simulink model "METI_TRAMI_Thermal_ver01_Jmaab_2018b_Intg"  (R2018b)
settings: Solver=ode8  StartTime=0  StopTime=end_time  FixedStep=sampling_time  RelTol=1e-3
PreLoadFcn:
  | METI_TRAMI_Thermal_ver01_Jmaab_PreLoad;
values from neighbouring files (symbols this model uses):
  degC2K = 273.15    [METI_TRAMI_Thermal_ver01_Jmaab_PreLoad.m]    (also in init_setting_METI.m)
  K2degC = -273.15    [METI_TRAMI_Thermal_ver01_Jmaab_PreLoad.m]    (also in init_setting_METI.m)
undefined symbols (not defined in the file or in its folder): ACC_D_Gain, ACC_I_Gain, ACC_P_Gain, ALT_CNT_ALT_OFF_RPM_HYS_rpm, ALT_CNT_ALT_ON_RPM_HYS_rpm, ALT_CNT_Alter_V_BASE_V, ALT_CNT_Alter_V_Kaisei_V, ALT_CNT_flag_disable_kaisei, ALT_CNT_V_Battely_Kudo_V, ALT_PNT_ALT_GDCurrent_A, ALT_PNT_ALT_GDVolt_V, ALT_PNT_Alter_limit_Current_V_table, ALT_PNT_Alter_limit_Current_V_table_x_rpm, ALT_PNT_Alter_trq_Nm_map, ALT_PNT_Alter_trq_Nm_map_x_rpm, ALT_PNT_Alter_trq_Nm_map_y_Current_A, ALT_PNT_Alter_trq_Nm_map_z_Volt_tgt_V, ALT_PNT_eta_pulley_alt, ALT_PNT_Gain_Alt_v_del, ALT_PNT_ratio_pulley_alt, ALT_PNT_Tau_Alternator_V_tgt_s, ALT_PNT_trq_alter_output_LL_Nm, BK_PNT_Pow_UL, BK_PNT_Tau_brake, Brk_LL, Brk_PGain, Brk_UL, BT_PNT_Lo_Capa_lo_batt_F, BT_PNT_Lo_ocv_SOC_lo_batt_OCV_V_table, BT_PNT_Lo_ocv_SOC_lo_batt_OCV_V_table_x_SOC, BT_PNT_Lo_R_lo_batt_ohm, BT_PNT_Lo_SOC_MAX_lo_batt, BT_PNT_Lo_SOC_MIN_lo_batt, BT_PNT_Lo_SOC_START_lo_batt, BT_PNT_Lo_V_start_ocv, DF_PNT_DF_gear, DF_PNT_DFBlock2DFAir_Heat_Resi_KpW, DF_PNT_DFBlock_Heat_Capa_JpK, DF_PNT_DFBlock_Temp_ini_degC, DF_PNT_DFOil2DFBlock_Heat_Resi_KpW, DF_PNT_DFOil_Heat_Capa_JpK, DF_PNT_DFOil_Temp_ini_degC, DF_PNT_Driveshaft_damper, DF_PNT_Driveshaft_delta_radps_LL, DF_PNT_Driveshaft_delta_radps_UL, DF_PNT_Driveshaft_spring, DF_PNT_eta_DF, DF_PNT_Outtemp_degC, DF_PNT_TMBlock2DFBlock_Heat_Resi_KpW, Driver_Brake_Const1, Driver_Brake_Const3, Driver_Brake_Switch_Const2, Driver_Brk_sh, drivmode_ACC, drivmode_CONST, drivmode_GensokuKaisei, drivmode_GensokuRikko, drivmode_STOP, EL_PNT_R_bodyelec_lo_ohm, ENG_CNT_acc_idlestop ... (+139)
libraries: METI_Lib_vehicle_model x33, simulink x7, AZAPA_Lib_vehicle_model x1
(part 4 of 4)

== system METI_TRAMI_Thermal_ver01_Jmaab_2018b_Intg/Driver/Driver_TRAMI/Driver2/Caliculate_Opeining_Accel/FF/Cal_M_ENG_jiku2 ==
  note: 軸トルクマップ
  FF_trq_accel_Nm : Inport
  pre_n_eng_rpm : Inport  Port=2
  2-D Lookup Table : Lookup_n-D  BreakpointsForDimension1=ENG_trq_rev  BreakpointsForDimension2=ENG_rpm  Table=ENG_throttle_rev  ExtrapMethod=Clip  UseLastTableValue=on  RndMeth=Simplest  InputSameDT=on
  2-D Lookup Table1 : Lookup_n-D  BreakpointsForDimension1=ENG_PNT_trq_Nm_map_y_throttle  BreakpointsForDimension2=ENG_PNT_trq_Nm_map_x_rpm  Table=ENG_PNT_trq_Nm_map  ExtrapMethod=Clip  UseLastTableValue=on  RndMeth=Simplest  InputSameDT=on
  Constant : Constant  Value=0
  Subsystem : Subsystem
  Sum : Sum  Inputs=|++
  FF_open_accel_per : Outport
  wires:
  FF_trq_accel_Nm/1 -> Sum/1
  2-D Lookup Table/1 -> Subsystem/1(In1)
  pre_n_eng_rpm/1 -> 2-D Lookup Table/2, 2-D Lookup Table1/2
  Constant/1 -> 2-D Lookup Table1/1
  Sum/1 -> 2-D Lookup Table/1
  2-D Lookup Table1/1 -> Sum/2
  Subsystem/1(Out1) -> FF_open_accel_per/1

== system METI_TRAMI_Thermal_ver01_Jmaab_2018b_Intg/Driver/Driver_TRAMI/Driver2/Caliculate_Opeining_Accel/FF/Inertial_Resistance ==
  V_tgt : Inport
  Constant : Constant  Value=M
  Derivative : Derivative
  Divide : Product  OutDataTypeStr=Inherit: Same as first input
  F_Inertia : Outport
  wires:
  Constant/1 -> Divide/2
  Derivative/1 -> Divide/1
  Divide/1 -> F_Inertia/1
  V_tgt/1 -> Derivative/1

== system METI_TRAMI_Thermal_ver01_Jmaab_2018b_Intg/Driver/Driver_TRAMI/Driver2/Caliculate_Opeining_Accel/FF/Rolling_Resistance ==
  note: 20151211修正
      |
      | 空気抵抗と表現を統一する、ため
      | -1のGainを削除
  V_tgt : Inport
  cal_roll_resi1 : METI_Lib_vehicle_model/vehicle_model/cal_roll_resi  Myu_tire=myu  Vehicle_Mass=M  Gravi_acc=g
      settings: SourceProductName=The database C:\Users\k-uekata\AppData\Roaming\MathWorks\MATLAB\R2018b\slblocks_master.db is locked, or a table in the database is locked. (database is locked)
  F_rollresi : Outport
  wires:
  V_tgt/1 -> cal_roll_resi1/1
  cal_roll_resi1/1 -> F_rollresi/1

== system METI_TRAMI_Thermal_ver01_Jmaab_2018b_Intg/Vehicle/CNT/ENG_CNT/ENG_Cntrl/Caliculate_Idle_Speed/Subsystem ==
  del_omg_engine : Inport
  flag_idle_fb : Inport  Port=2
  Gain : Gain  Gain=ENG_CNT_gain_p_per_isc
  Logical Operator1 : Logic  Operator=NOT  AllPortsSameDT=off  OutDataTypeStr=boolean
  Memory : Memory  InitialCondition=4
  Saturation : Saturate  UpperLimit=ENG_CNT_per_isc_max  LowerLimit=ENG_CNT_per_isc_min
  Switch : Switch  Criteria=u2 > Threshold  Threshold=0.5
  per_isc_[%] : Outport
  wires:
  Logical Operator1/1 -> Switch/2
  del_omg_engine/1 -> Gain/1
  Saturation/1 -> Memory/1, per_isc_[%]/1
  Memory/1 -> Switch/1
  Gain/1 -> Switch/3
  flag_idle_fb/1 -> Logical Operator1/1
  Switch/1 -> Saturation/1

== system METI_TRAMI_Thermal_ver01_Jmaab_2018b_Intg/Vehicle/CNT/ENG_CNT/ENG_Cntrl/Caliculate_Idle_Speed/Subsystem1 ==
  note: アイドル回転数時のFB
  omg_tgt_idle : Inport
  n_eng_rpm : Inport  Port=2
  per_throttle_base : Inport  Port=3
  flag_Lockup : Inport  Port=4
  flag_IdleStop : Inport  Port=5
  Logical Operator : Logic  Operator=OR  AllPortsSameDT=off  OutDataTypeStr=boolean
  Logical Operator1 : Logic  Operator=NOT  AllPortsSameDT=off  OutDataTypeStr=boolean
  Logical Operator2 : Logic  Inputs=3  AllPortsSameDT=off  OutDataTypeStr=boolean
  Logical Operator3 : Logic  Operator=NOT  AllPortsSameDT=off  OutDataTypeStr=boolean
  Logical Operator4 : Logic  Operator=NOT  AllPortsSameDT=off  OutDataTypeStr=boolean
  Logical Operator5 : Logic  AllPortsSameDT=off  OutDataTypeStr=boolean
  Relational Operator : RelationalOperator  Operator=<  OutDataTypeStr=boolean  RndMeth=Nearest
  Relational Operator2 : RelationalOperator  Operator=>  OutDataTypeStr=boolean  RndMeth=Nearest
  per_throttle_isc_fb : Constant  Value=ENG_CNT_per_throttle_isc_fb
  flag_idle_fb : Outport
  wires:
  Logical Operator/1 -> flag_idle_fb/1
  Logical Operator4/1 -> Logical Operator5/2
  flag_IdleStop/1 -> Logical Operator4/1
  n_eng_rpm/1 -> Relational Operator2/2
  omg_tgt_idle/1 -> Relational Operator2/1
  Logical Operator2/1 -> Logical Operator/1
  Logical Operator3/1 -> Logical Operator2/3
  flag_Lockup/1 -> Logical Operator3/1
  Logical Operator5/1 -> Logical Operator/2
  Logical Operator1/1 -> Logical Operator2/2
  Relational Operator/1 -> Logical Operator5/1, Logical Operator1/1
  Relational Operator2/1 -> Logical Operator2/1
  per_throttle_isc_fb/1 -> Relational Operator/2
  per_throttle_base/1 -> Relational Operator/1

== system METI_TRAMI_Thermal_ver01_Jmaab_2018b_Intg/Vehicle/CNT/TM_CNT/TM_CNT/TM_CNT/TM_Ctrl ==
  v_VL_PNT_kmph : Inport
  n_TM_PNT_rpm : Inport  Port=2
  T_TMTH_PNT_CVTF_degC : Inport  Port=3
  T_ENGTH_PNT_Coolant_degC : Inport  Port=4
  open_throttle_per : Inport  Port=5
  CVT_ECU : Subsystem
  K->degC : Subsystem  Commented=through
  K->degC1 : Subsystem  Commented=through
  LockupClutch_ECU : Subsystem
  Memory{,1..4} (5 alike) : Memory  Commented=through
  Signal Specification : SignalSpecification
  Signal Specification1 : SignalSpecification
  WarmerECU : Subsystem
  flag_Lockup : Outport
  omg_Slip_rpm : Outport  Port=2
  ratio_CVT : Outport  Port=3
  R_CVTF_warmer_tgt_KpW : Outport  Port=4
  tag scope: tScope_CVTratio=scoped, tScope_Luckup=scoped
  wires:
  CVT_ECU/1(ratio_CVT) -> Signal Specification1/1, ratio_CVT/1  "ratio_CVT"
  LockupClutch_ECU/1(flag_Lockup) -> Signal Specification/1, flag_Lockup/1  "flag_Lockup"
  LockupClutch_ECU/2(omg_Slip_rpm) -> omg_Slip_rpm/1  "omg_Slip_rpm"
  open_throttle_per/1 -> Memory1/1
  Memory/1 -> LockupClutch_ECU/1(v_vehicle)
  Memory1/1 -> CVT_ECU/1(per_throttle), LockupClutch_ECU/2(per_throttle)
  Memory2/1 -> CVT_ECU/2(omg_pera)
  n_TM_PNT_rpm/1 -> Memory2/1
  v_VL_PNT_kmph/1 -> Memory/1
  T_TMTH_PNT_CVTF_degC/1 -> Memory3/1
  T_ENGTH_PNT_Coolant_degC/1 -> Memory4/1
  Memory3/1 -> K->degC/1(K)
  Memory4/1 -> K->degC1/1(K)
  WarmerECU/1(R_CVTF_warmer_tgt_KpW) -> R_CVTF_warmer_tgt_KpW/1  "R_CVTF_warmer_tgt_KpW"
  K->degC/1(degC) -> WarmerECU/1(T_TMTH_PNT_CVTF_dC)
  K->degC1/1(degC) -> WarmerECU/2(T_ENG_Coolant_dC)
  Signal Specification/1 -> [tScope_Luckup]  "tScope_Luckup"
  Signal Specification1/1 -> [tScope_CVTratio]  "tScope_CVTratio"

== system METI_TRAMI_Thermal_ver01_Jmaab_2018b_Intg/Vehicle/PTTH/DTTH_PNT/DTTH_PNT/DTTH_PNT/DFTH_PNT ==
  note: T/Mブロックから
      | 受け取る熱量
  note: DFオイルの
      | 熱容量
  note: DFブロックの
      | 熱容量
  note: DFの損失が
      | DFオイルへの熱量
  note: エネルギーの
      | 向きの定義（仮）
      | →→→
  note: エネルギーの
      | 向きの定義（仮）
      | →→→
  note: エネルギーの
      | 向きの定義（仮）
      | →→→
  note: エネルギーの
      | 向きの定義（仮）
      | →→→
  note: エネルギーの
      | 向きの定義（仮）
      | →→→
  T_DF_Block_K : Inport
  PHI_DF_PNT_W : Inport  Port=2
  T_ATM_PNT_DF_K : Inport  Port=3
  DFBlock_Heat_Capacity : Subsystem
  DFOil2DFBlock_Heat_Resistance : Subsystem
  DFOil_Heat_Capacity : Subsystem
  ENGBlock2Air_Heat_Resistance : Subsystem
  TMBlock2DFBlock_Heat_Resistance : Subsystem
  Terminator : Terminator
  PHI_DF_Block_W : Outport
  PHI_DFTH_PNT_W : Outport  Port=2
  T_DFBlock_K : Outport  Port=3
  wires:
  DFOil_Heat_Capacity/1(T_DFOil2_K) -> DFOil2DFBlock_Heat_Resistance/1(T_DFOil_Resi2_K)
  DFOil2DFBlock_Heat_Resistance/1(PHI_DFOil_Resi2_W) -> DFOil_Heat_Capacity/1(PHI_DFOil2_W)
  DFBlock_Heat_Capacity/3(T_DFBlock1_K) -> DFOil2DFBlock_Heat_Resistance/2(T_DFBlock_Resi_K)
  DFOil2DFBlock_Heat_Resistance/2(PHI_DFBlock_Resi_W) -> DFBlock_Heat_Capacity/3(PHI_DFBlock1_W)
  ENGBlock2Air_Heat_Resistance/1(PHI_DFBlock_Resi_W) -> DFBlock_Heat_Capacity/1(PHI_DFBlock3_W)
  DFBlock_Heat_Capacity/2(T_DFBlock3_K) -> ENGBlock2Air_Heat_Resistance/1(T_DFBlock_Resi_K)
  T_ATM_PNT_DF_K/1 -> ENGBlock2Air_Heat_Resistance/2(T_DF_Air_Resi_K)
  ENGBlock2Air_Heat_Resistance/2(PHI_DF_Air_Resi_W) -> PHI_DFTH_PNT_W/1  "PHI_DFTH_PNT_W"
  T_DF_Block_K/1 -> TMBlock2DFBlock_Heat_Resistance/2(T_TMBlock_Resi_K)
  TMBlock2DFBlock_Heat_Resistance/2(PHI_TMBlock_Resi_W) -> PHI_DF_Block_W/1  "PHI_DF_Block_W"
  TMBlock2DFBlock_Heat_Resistance/1(PHI_DFBlock_Resi_W) -> DFBlock_Heat_Capacity/2(PHI_DFBlock2_W)
  DFBlock_Heat_Capacity/1(T_DFBlock2_K) -> T_DFBlock_K/1, TMBlock2DFBlock_Heat_Resistance/1(T_DFBlock_Resi_K)  "T_DFBlock_K"
  DFOil_Heat_Capacity/2(T_DFOil1_K) -> Terminator/1
  PHI_DF_PNT_W/1 -> DFOil_Heat_Capacity/2(PHI_DFOil1_W)

== system METI_TRAMI_Thermal_ver01_Jmaab_2018b_Intg/Vehicle/PTTH/DTTH_PNT/DTTH_PNT/DTTH_PNT/TMTH_PNT ==
  note: CVTFの
      | 熱容量
  note: T/Mブロックの
      | 熱容量
  note: DFブロックへ
      | 放熱する熱量
  note: エンジンブロックから
      | 受け取る熱量
  note: CVTFからエンジン冷却水へ
      | 放熱する熱量
  note: T/Mの入力-出力が
      | CVTFへの熱量
  note: エネルギーの
      | 向きの定義（仮）
      | ←←←
  note: エネルギーの
      | 向きの定義（仮）
      | →→→
  note: エネルギーの
      | 向きの定義（仮）
      | →→→
  note: エネルギーの
      | 向きの定義（仮）
      | →→→
  note: エネルギーの
      | 向きの定義（仮）
      | →→→
  note: エネルギーの
      | 向きの定義（仮）
      | →→→
  note: エネルギーの
      | 向きの定義（仮）
      | →→→
  note: TMブロックからから大気へ
      | 放熱する熱量
  W_TM_Block0_W : Inport
  R_CVTF_warmer_tgt_KpW : Inport  Port=2
  PHI_TM_PNT_W : Inport  Port=3
  T_TM_Block_Resi_K : Inport  Port=4
  T_ENGTH_PNT_Coolant_K : Inport  Port=5
  T_ATM_PNT_TM_K : Inport  Port=6
  CVTF2Coolant_Heat_Resistance : Subsystem
  CVTF2TMBlock_Heat_Resistance : Subsystem
  CVTF_Heat_Capacity : Subsystem
  ENGBlock2TMBlock_Heat_Resistance : Subsystem
  Goto : Goto  Commented=on  GotoTag=R_CVTF_warmer_tgt_KpW  TagVisibility=global
  TMBlock2Air_Heat_Resistance : Subsystem
  TMBlock_Heat_Capacity : Subsystem
  T_TMTH_PNT_CVTF1_K : Outport
  T_TM_Block0_K : Outport  Port=2
  PHI_TM_CVTF_Resi_W : Outport  Port=3
  T_TMTH_PNT_CVTF_K : Outport  Port=4
  PHI_ENGBlock_Resi2_W : Outport  Port=5
  PHI_TMTH_PNT_W : Outport  Port=6
  wires:
  CVTF_Heat_Capacity/1(T_CVTF4_K) -> CVTF2TMBlock_Heat_Resistance/1(T_CVTF_Resi4_K)
  CVTF2TMBlock_Heat_Resistance/1(PHI_CVTF_Resi4_W) -> CVTF_Heat_Capacity/1(PHI_CVTF4_W)
  TMBlock_Heat_Capacity/4(T_TMBlock1_K) -> CVTF2TMBlock_Heat_Resistance/2(T_TMBlock_Resi1_K)
  CVTF2TMBlock_Heat_Resistance/2(PHI_TMBlock_Resi1_W) -> TMBlock_Heat_Capacity/3(PHI_TMBlock1_W)
  CVTF_Heat_Capacity/3(T_CVTF1_K) -> T_TMTH_PNT_CVTF_K/1, T_TMTH_PNT_CVTF1_K/1  "T_TMTH_PNT_CVTF_K"
  PHI_TM_PNT_W/1 -> CVTF_Heat_Capacity/2(PHI_CVTF1_W)
  TMBlock2Air_Heat_Resistance/1(PHI_TMBlock_Resi3_W) -> TMBlock_Heat_Capacity/1(PHI_TMBlock3_W)
  TMBlock_Heat_Capacity/2(T_TMBlock3_K) -> TMBlock2Air_Heat_Resistance/1(T_TMBlock_Resi3_K)
  T_ATM_PNT_TM_K/1 -> TMBlock2Air_Heat_Resistance/2(T_TM_Air_Resi1_K)
  TMBlock2Air_Heat_Resistance/2(PHI_TM_Air_Resi1_W) -> PHI_TMTH_PNT_W/1  "PHI_TMTH_PNT_W"
  T_TM_Block_Resi_K/1 -> ENGBlock2TMBlock_Heat_Resistance/2(T_ENGBlock_Resi2_K)
  ENGBlock2TMBlock_Heat_Resistance/2(PHI_ENGBlock_Resi2_W) -> PHI_ENGBlock_Resi2_W/1  "PHI_ENGBlock_Resi2_W"
  CVTF_Heat_Capacity/2(T_CVTF2_K) -> CVTF2Coolant_Heat_Resistance/1(T_CVTF_Resi2_K)
  CVTF2Coolant_Heat_Resistance/2(PHI_CVTF_Resi2_W) -> CVTF_Heat_Capacity/3(PHI_CVT2_W)
  CVTF2Coolant_Heat_Resistance/1(PHI_Coolant_Resi2_W) -> PHI_TM_CVTF_Resi_W/1  "PHI_TM_CVTF_Resi_W"
  T_ENGTH_PNT_Coolant_K/1 -> CVTF2Coolant_Heat_Resistance/3(T_Coolant_Resi2_K)
  ENGBlock2TMBlock_Heat_Resistance/1(PHI_TMBlock_Resi2_W) -> TMBlock_Heat_Capacity/2(PHI_TMBlock2_W)
  TMBlock_Heat_Capacity/1(T_TMBlock2_K) -> ENGBlock2TMBlock_Heat_Resistance/1(T_TMBlock_Resi2_K)
  TMBlock_Heat_Capacity/3(T_TMBlock4_K) -> T_TM_Block0_K/1  "T_TM_Block0_degC"
  W_TM_Block0_W/1 -> TMBlock_Heat_Capacity/4(PHI_TMBlock4_W)
  R_CVTF_warmer_tgt_KpW/1 -> CVTF2Coolant_Heat_Resistance/2(R_CVTF_warmer_tgt_KpW), Goto/1

== system METI_TRAMI_Thermal_ver01_Jmaab_2018b_Intg/Vehicle/PTTH/ENGTH_PNT/ENGTH/Coolant_Heat_Capacity/degC->K ==
  degC : Inport
  Constant2 : Constant  Value=degC2K
  Sum : Sum  Inputs=++|
  K : Outport
  wires:
  degC/1 -> Sum/2
  Constant2/1 -> Sum/1
  Sum/1 -> K/1

== system METI_TRAMI_Thermal_ver01_Jmaab_2018b_Intg/Vehicle/PTTH/ENGTH_PNT/ENGTH/ENGBlock_Heat_Capacity/degC->K ==
  degC : Inport
  Constant2 : Constant  Value=degC2K
  Sum : Sum  Inputs=++|
  K : Outport
  wires:
  degC/1 -> Sum/2
  Constant2/1 -> Sum/1
  Sum/1 -> K/1

== system METI_TRAMI_Thermal_ver01_Jmaab_2018b_Intg/Vehicle/PTTH/ENGTH_PNT/ENGTH/ENGOil_Heat_Capacity/degC->K ==
  degC : Inport
  Constant2 : Constant  Value=degC2K
  Sum : Sum  Inputs=++|
  K : Outport
  wires:
  degC/1 -> Sum/2
  Constant2/1 -> Sum/1
  Sum/1 -> K/1

== system METI_TRAMI_Thermal_ver01_Jmaab_2018b_Intg/Vehicle/PTTH/ENGTH_PNT/ENGTH/ENGOil_Heat_Capacity1/degC->K ==
  degC : Inport
  Constant2 : Constant  Value=degC2K
  Sum : Sum  Inputs=++|
  K : Outport
  wires:
  degC/1 -> Sum/2
  Constant2/1 -> Sum/1
  Sum/1 -> K/1

== system METI_TRAMI_Thermal_ver01_Jmaab_2018b_Intg/Vehicle/PTTH/RDTH_PNT/RDTH/ENGBlock2Coolant_Heat_Resistance/K->degC ==
  K : Inport
  Constant2 : Constant  Value=K2degC
  Sum : Sum  Inputs=++|
  degC : Outport
  wires:
  K/1 -> Sum/2
  Constant2/1 -> Sum/1
  Sum/1 -> degC/1

== system METI_TRAMI_Thermal_ver01_Jmaab_2018b_Intg/Vehicle/PTTH/RDTH_PNT/RDTH/RDCoolant_Heat_Capacity/degC->K ==
  degC : Inport
  Constant2 : Constant  Value=degC2K
  Sum : Sum  Inputs=++|
  K : Outport
  wires:
  degC/1 -> Sum/2
  Constant2/1 -> Sum/1
  Sum/1 -> K/1

== system METI_TRAMI_Thermal_ver01_Jmaab_2018b_Intg/Vehicle/TM_PNT/TM_PNT/TM_PNT/DF_PNT/DriveShaft ==
  note: ドライブシャフトモデル
      | 硬いバネダンパー
  w_TR_PNT_radps : Inport
  w_DS_PNT_in_radps : Inport  Port=2
  Gain : Gain  Gain=-1
  Gain1 : Gain  Gain=DF_PNT_Driveshaft_spring
  Gain2 : Gain  Gain=DF_PNT_Driveshaft_damper
  Integrator : Integrator  LimitOutput=on  UpperSaturationLimit=DF_PNT_Driveshaft_delta_radps_UL  LowerSaturationLimit=DF_PNT_Driveshaft_delta_radps_LL
  Sum : Sum  Inputs=|+-
  Sum2 : Sum  Inputs=|++
  trq_DS_PNT_in_Nm : Outport
  trq_DF_PNT_Nm : Outport  Port=2
  wires:
  w_TR_PNT_radps/1 -> Sum/2
  w_DS_PNT_in_radps/1 -> Sum/1
  Integrator/1 -> Gain1/1
  Sum/1 -> Integrator/1, Gain2/1
  Gain1/1 -> Sum2/1
  Gain2/1 -> Sum2/2
  Sum2/1 -> Gain/1, trq_DS_PNT_in_Nm/1
  Gain/1 -> trq_DF_PNT_Nm/1

== system METI_TRAMI_Thermal_ver01_Jmaab_2018b_Intg/Vehicle/TM_PNT/TM_PNT/TM_PNT/TM_PNT/Flywheel ==
  trq_TM_PNT_in_Nm : Inport
  trq_TM_PNT_in_Nm1 : Inport  Port=2
  Divide : Product  Inputs=*/
  Inertia : Constant  Value=TM_PNT_Flywheel_Inertia_kgm2
  Integrator : Integrator  InitialCondition=TM_PNT_Flywheel_Init_radps  LimitOutput=on  LowerSaturationLimit=0
  P_cal : METI_Lib_vehicle_model/P_cal  Commented=on  Type_energy=回転運動  Type_output_energy=出力  Power_name=Po_  t_Workspace_Name=TM_PNT_Flywheel  P_VariableName=Po_TM_PNT_Flywheel  Across_VariableName=w_TM_PNT_Flywheel  Throgh_VariableName=tq_TM_PNT_Flywheel
  Sum : Sum  Inputs=|++
  Terminator : Terminator  Commented=on
  w_ENG_PNT_radps : Outport
  w_TM_PNT_in_radps : Outport  Port=2
  wires:
  Integrator/1 -> P_cal/1, w_TM_PNT_in_radps/1, w_ENG_PNT_radps/1
  trq_TM_PNT_in_Nm/1 -> Sum/1
  trq_TM_PNT_in_Nm1/1 -> Sum/2
  Inertia/1 -> Divide/2
  Sum/1 -> Divide/1, P_cal/2
  P_cal/1 -> Terminator/1
  Divide/1 -> Integrator/1

== system METI_TRAMI_Thermal_ver01_Jmaab_2018b_Intg/Vehicle/TM_PNT/TM_PNT/TM_PNT/TM_PNT/Inertia ==
  trq_TM_PNT_out_Nm0 : Inport
  trq_TM_PNT_Nm : Inport  Port=2
  Divide : Product  Inputs=*/
  Inertia : Constant  Value=TM_PNT_Driveshaft_Inertia_kgm2
  Integrator : Integrator  InitialCondition=000*(2*pi)/60  LimitOutput=on  LowerSaturationLimit=0
  P_cal : METI_Lib_vehicle_model/P_cal  Type_energy=回転運動  Type_output_energy=出力  Power_name=Po_  t_Workspace_Name=TM_PNT_inertia_MECK  P_VariableName=Po_TM_PNT_inertia_MECK  Across_VariableName=w_TM_PNT_inertia_MECK  Throgh_VariableName=tq_TM_PNT_inertia_MECK
  Sum : Sum  Inputs=|++
  Terminator : Terminator
  w_TM_PNT_out_radps : Outport
  w_TM_PNT_out_radps0 : Outport  Port=2
  wires:
  Integrator/1 -> P_cal/1, w_TM_PNT_out_radps0/1, w_TM_PNT_out_radps/1
  Divide/1 -> Integrator/1
  trq_TM_PNT_out_Nm0/1 -> Sum/1
  trq_TM_PNT_Nm/1 -> Sum/2
  Inertia/1 -> Divide/2
  Sum/1 -> Divide/1, P_cal/2
  P_cal/1 -> Terminator/1

== system METI_TRAMI_Thermal_ver01_Jmaab_2018b_Intg/Vehicle/TM_PNT/TM_PNT/TM_PNT/TM_PNT/K->degC6 ==
  K : Inport
  Constant2 : Constant  Value=K2degC
  Sum : Sum  Inputs=++|
  degC : Outport
  wires:
  K/1 -> Sum/2
  Constant2/1 -> Sum/1
  Sum/1 -> degC/1

== system METI_TRAMI_Thermal_ver01_Jmaab_2018b_Intg/Vehicle/TM_PNT/TM_PNT/TM_PNT/TM_PNT/TC_PNT ==
  note: ロックアップクラッチ
  note: トルクコンバータ
  flag_Lockup : Inport
  omg_Slip_rpm : Inport  Port=2
  w_TM_PNT_in_radps : Inport  Port=3
  w_TM_PNT_in_radps2 : Inport  Port=4
  Gain : Gain  Gain=-1
  LU_Clutch : Subsystem
  P_cal : METI_Lib_vehicle_model/P_cal  Type_energy=回転運動  Type_output_energy=出力  Power_name=Po_  t_Workspace_Name=TM_PNT_TC_MECK_UP  P_VariableName=Po_TM_PNT_TC_MECK_UP  Across_VariableName=w_TM_PNT_TC_MECK_UP  Throgh_VariableName=tq_TM_PNT_TC_MECK_UP
  P_cal1 : METI_Lib_vehicle_model/P_cal  Type_energy=回転運動  Type_output_energy=出力  Power_name=Po_  t_Workspace_Name=TM_PNT_TC_MECK_DN  P_VariableName=Po_TM_PNT_TC_MECK_DN  Across_VariableName=w_TM_PNT_TC_MECK_DN  Throgh_VariableName=tq_TM_PNT_TC_MECK_DN
  P_cal2 : METI_Lib_vehicle_model/P_cal  Type_energy=回転運動  Type_output_energy=出力  Power_name=Po_  t_Workspace_Name=TM_PNT_LU_MECK_UP  P_VariableName=Po_TM_PNT_LU_MECK_UP  Across_VariableName=w_TM_PNT_LU_MECK_UP  Throgh_VariableName=tq_TM_PNT_LU_MECK_UP
  P_cal3 : METI_Lib_vehicle_model/P_cal  Type_energy=回転運動  Type_output_energy=出力  Power_name=Po_  t_Workspace_Name=TM_PNT_LU_MECK_DN  P_VariableName=Po_TM_PNT_LU_MECK_DN  Across_VariableName=w_TM_PNT_LU_MECK_DN  Throgh_VariableName=tq_TM_PNT_LU_MECK_DN
  Sum : Sum  Inputs=|++
  Sum1 : Sum  Inputs=|++
  T_C : Subsystem
  Terminator{,1..4} (5 alike) : Terminator
  trq_TM_PNT_in_Nm2 : Outport
  trq_TM_PNT_in_Nm1 : Outport  Port=2
  wires:
  T_C/2(trq_TC_Nm2) -> Sum/2, P_cal/2
  w_TM_PNT_in_radps/1 -> T_C/1(w_TM_PNT_in_radps1), P_cal/1, LU_Clutch/2(w_TM_PNT_in_radps1), P_cal2/1
  Sum/1 -> Gain/1
  T_C/1(trq_TC_Nm1) -> P_cal1/2, Sum1/2
  Sum1/1 -> trq_TM_PNT_in_Nm2/1
  w_TM_PNT_in_radps2/1 -> LU_Clutch/3(w_TM_PNT_in_radps2), P_cal1/1, P_cal3/1, T_C/2(w_TM_PNT_in_radps2)
  P_cal/1 -> Terminator/1
  P_cal1/1 -> Terminator1/1
  omg_Slip_rpm/1 -> Terminator3/1
  LU_Clutch/1(trq_LUC_Nm1) -> Sum/1, P_cal2/2
  LU_Clutch/2(trq_LUC_Nm2) -> Sum1/1, P_cal3/2
  flag_Lockup/1 -> LU_Clutch/1(LockUP_Signal)
  P_cal2/1 -> Terminator2/1
  P_cal3/1 -> Terminator4/1
  Gain/1 -> trq_TM_PNT_in_Nm1/1

== system METI_TRAMI_Thermal_ver01_Jmaab_2018b_Intg/Vehicle/TM_PNT/TM_PNT/TM_PNT/TM_PNT/VR_PNT ==
  note: ギア比変換
  ratio_CVT : Inport
  trq_TM_PNT_in_Nm2 : Inport  Port=2
  w_TM_PNT_out_radps0 : Inport  Port=3
  T_TMTH_PNT_CVTF_dC : Inport  Port=4
  1-D Lookup Table : Lookup_n-D  NumberOfTableDimensions=1  BreakpointsForDimension1=TM_PNT_eta_CVT_x_CVTF_degC  Table=TM_PNT_eta_CVT  ExtrapMethod=Clip  InternalRulePriority=Speed  RndMeth=Simplest  InputSameDT=on
  Goto1 : Goto  Commented=on  GotoTag=trq_Variator_Nm
  P_cal : METI_Lib_vehicle_model/P_cal  Type_energy=回転運動  Type_output_energy=損失  Power_name=Pl_  t_Workspace_Name=TM_PNT_Variator_MECK_LOSS  P_VariableName=Pl_TM_PNT_Variator_MECK_LOSS  Across_VariableName=w_TM_PNT_Variator_MECK_LOSS  Throgh_VariableName=tq_TM_PNT_Variator_MECK_LOSS
  Product : Product  RndMeth=Zero
  Product1 : Product  RndMeth=Zero
  Transfer Fcn : TransferFcn  Denominator=[TM_PNT_Tau_CVT_ratio_s 1]
  eta_cal_CVT : METI_Lib_vehicle_model/eta_cal_InHi  SystemSampleTime=-1
  trq_TM_PNT_out_Nm0 : Outport
  w_TM_PNT_in_radps2 : Outport  Port=2
  tag scope: tScope_CVTLoss=scoped
  wires:
  trq_TM_PNT_in_Nm2/1 -> eta_cal_CVT/2
  Product/1 -> w_TM_PNT_in_radps2/1, P_cal/1
  w_TM_PNT_out_radps0/1 -> Product/2
  ratio_CVT/1 -> Transfer Fcn/1
  Product1/1 -> Goto1/1, trq_TM_PNT_out_Nm0/1
  eta_cal_CVT/2 -> Product1/2
  P_cal/1 -> [tScope_CVTLoss]  "tScope_CVTLoss"
  Transfer Fcn/1 -> Product1/1, Product/1
  1-D Lookup Table/1 -> eta_cal_CVT/1  "TM_eta"
  eta_cal_CVT/1 -> P_cal/2
  T_TMTH_PNT_CVTF_dC/1 -> 1-D Lookup Table/1

== system METI_TRAMI_Thermal_ver01_Jmaab_2018b_Intg/Driver/Driver/Driver/Caliculate_Opeining_Accel/FF/Cal_M_ENG_jiku2/Subsystem ==
  In1 : Inport
  Constant1 : Constant  Value=0
  Switch : Switch  Criteria=u2 > Threshold  Threshold=0.1
  Out1 : Outport
  wires:
  Switch/1 -> Out1/1
  Constant1/1 -> Switch/3
  In1/1 -> Switch/2, Switch/1

== system METI_TRAMI_Thermal_ver01_Jmaab_2018b_Intg/Driver/Driver_TRAMI/Driver2/Caliculate_Opeining_Accel/FF/Cal_M_ENG_jiku2/Subsystem ==
  In1 : Inport
  Constant1 : Constant  Value=0
  Switch : Switch  Criteria=u2 > Threshold  Threshold=0.1
  Out1 : Outport
  wires:
  Switch/1 -> Out1/1
  Constant1/1 -> Switch/3
  In1/1 -> Switch/2, Switch/1

== system METI_TRAMI_Thermal_ver01_Jmaab_2018b_Intg/Vehicle/CNT/TM_CNT/TM_CNT/TM_CNT/TM_Ctrl/CVT_ECU ==
  per_throttle : Inport
  omg_pera : Inport  Port=2
  1-D Lookup Table : Lookup_n-D  NumberOfTableDimensions=1  BreakpointsForDimension1=TM_CNT_CVTpritgt_rpm_table_x_TVO  Table=TM_CNT_CVTpritgt_rpm_table  RndMeth=Simplest  InputSameDT=on
  Constant2 : Constant  Value=TM_CNT_CVT_radpmin_min_rpm
  Divide : Product  Inputs=*/
  Gain2 : Gain  Gain=TM_CNT_Gain_CVT_ECU
  HighestRatio : Constant  Value=TM_CNT_CVT_ratio_LL
  LowestRatio : Constant  Value=TM_CNT_CVT_ratio_UL
  MinMax : MinMax  Function=max  Inputs=2
  Saturation : Saturate  UpperLimit=TM_CNT_delta_CVT_ratio_UL  LowerLimit=TM_CNT_delta_CVT_ratio_LL
  Saturation Dynamic : simulink/Discontinuities/Saturation Dynamic  OutMin=[]  OutMax=[]  OutDataTypeStr=Inherit: Same as second input  OutDataType=fixdt(1, 16)  OutScaling=2^-10  DoSatur=off
  Sum : Sum  Inputs=|+-
  Sum1 : Sum  Inputs=|++
  Unit Delay : UnitDelay  InitialCondition=1  SampleTime=-1
  ratio_CVT : Outport
  wires:
  1-D Lookup Table/1 -> Divide/1
  Divide/1 -> Saturation Dynamic/2
  LowestRatio/1 -> Saturation Dynamic/1
  HighestRatio/1 -> Saturation Dynamic/3
  MinMax/1 -> Divide/2
  Saturation Dynamic/1 -> Sum/1
  Unit Delay/1 -> Sum1/2, Sum/2
  Sum1/1 -> ratio_CVT/1, Unit Delay/1
  Sum/1 -> Gain2/1
  Gain2/1 -> Saturation/1
  per_throttle/1 -> 1-D Lookup Table/1
  omg_pera/1 -> MinMax/2
  Saturation/1 -> Sum1/1
  Constant2/1 -> MinMax/1

== system METI_TRAMI_Thermal_ver01_Jmaab_2018b_Intg/Vehicle/CNT/TM_CNT/TM_CNT/TM_CNT/TM_Ctrl/K->degC ==
  K : Inport
  Constant2 : Constant  Value=K2degC
  Sum : Sum  Inputs=++|
  degC : Outport
  wires:
  Sum/1 -> degC/1
  Constant2/1 -> Sum/1
  K/1 -> Sum/2

== system METI_TRAMI_Thermal_ver01_Jmaab_2018b_Intg/Vehicle/CNT/TM_CNT/TM_CNT/TM_CNT/TM_Ctrl/K->degC1 ==
  K : Inport
  Constant2 : Constant  Value=K2degC
  Sum : Sum  Inputs=++|
  degC : Outport
  wires:
  K/1 -> Sum/2
  Constant2/1 -> Sum/1
  Sum/1 -> degC/1

== system METI_TRAMI_Thermal_ver01_Jmaab_2018b_Intg/Vehicle/CNT/TM_CNT/TM_CNT/TM_CNT/TM_Ctrl/LockupClutch_ECU ==
  v_vehicle : Inport
  per_throttle : Inport  Port=2
  2-D Lookup Table : Lookup_n-D  BreakpointsForDimension1=TM_CNT_LU_slip_rpm_map_y_TVO  BreakpointsForDimension2=TM_CNT_LU_slip_rpm_map_x_speed_kmph  Table=TM_CNT_LU_slip_rpm_map  RndMeth=Simplest  InputSameDT=on
  Relay : Relay  OnSwitchValue=TM_CNT_LU_Clutch_RelayON_rpm  OffSwitchValue=TM_CNT_LU_Clutch_RelayOFF_rpm  OnOutputValue=0  OffOutputValue=1
  flag_Lockup : Outport
  omg_Slip_rpm : Outport  Port=2
  wires:
  v_vehicle/1 -> 2-D Lookup Table/2
  2-D Lookup Table/1 -> omg_Slip_rpm/1, Relay/1
  per_throttle/1 -> 2-D Lookup Table/1
  Relay/1 -> flag_Lockup/1

== system METI_TRAMI_Thermal_ver01_Jmaab_2018b_Intg/Vehicle/CNT/TM_CNT/TM_CNT/TM_CNT/TM_Ctrl/WarmerECU ==
  note: ENG冷却水温＞CVTF温度
      | の時にこのマップを使用する
  note: CVTF温度が熱い時に
      | このマップを使用する
  T_TMTH_PNT_CVTF_dC : Inport
  T_ENG_Coolant_dC : Inport  Port=2
  1-D Lookup Table1 : Lookup_n-D  NumberOfTableDimensions=1  BreakpointsForDimension1=TM_CNT_CVTFwarmer_KpW_x_T_ENGCoolant  BeginIndexSearchUsingPreviousIndexResult=on  Table=TM_CNT_CVTFwarmer_KpW  ExtrapMethod=Clip  InternalRulePriority=Speed  RndMeth=Simplest  InputSameDT=on
  1-D Lookup Table2 : Lookup_n-D  NumberOfTableDimensions=1  BreakpointsForDimension1=TM_CNT_CVTFwarmer2_KpW_x_T_CVTF  BeginIndexSearchUsingPreviousIndexResult=on  Table=TM_CNT_CVTFwarmer2_KpW  ExtrapMethod=Clip  InternalRulePriority=Speed  RndMeth=Simplest  InputSameDT=on
  Add1 : Sum  Inputs=+-
  Compare To Zero1 : simulink/Logic and Bit Operations/Compare To Zero  relop=>  OutDataTypeStr=boolean
  Constant1 : Constant  Value=TM_CNT_CVTFwarmer_cold_Coolant_KpW
  MinMax : MinMax  Inputs=2
  Switch1 : Switch  Criteria=u2 > Threshold
  R_CVTF_warmer_tgt_KpW : Outport
  wires:
  MinMax/1 -> R_CVTF_warmer_tgt_KpW/1
  Add1/1 -> Compare To Zero1/1
  Compare To Zero1/1 -> Switch1/2
  1-D Lookup Table1/1 -> Switch1/1
  Constant1/1 -> Switch1/3
  T_ENG_Coolant_dC/1 -> 1-D Lookup Table1/1, Add1/1
  T_TMTH_PNT_CVTF_dC/1 -> 1-D Lookup Table2/1, Add1/2
  Switch1/1 -> MinMax/1
  1-D Lookup Table2/1 -> MinMax/2

== system METI_TRAMI_Thermal_ver01_Jmaab_2018b_Intg/Vehicle/PTTH/DTTH_PNT/DTTH_PNT/DTTH_PNT/DFTH_PNT/DFBlock_Heat_Capacity ==
  PHI_DFBlock3_W : Inport
  PHI_DFBlock2_W : Inport  Port=2
  PHI_DFBlock1_W : Inport  Port=3
  Add : Sum  Inputs=+++
  Add1 : Sum
  Constant : Constant  Value=DF_PNT_DFBlock_Heat_Capa_JpK
  Constant1 : Constant  Value=DF_PNT_DFBlock_Temp_ini_degC
  Divide : Product  Inputs=/*
  Integrator : Integrator
  degC->K : Subsystem
  T_DFBlock2_K : Outport
  T_DFBlock3_K : Outport  Port=2
  T_DFBlock1_K : Outport  Port=3
  wires:
  PHI_DFBlock1_W/1 -> Add/1
  Constant/1 -> Divide/1
  Add/1 -> Divide/2
  Divide/1 -> Integrator/1
  Integrator/1 -> Add1/2
  Add1/1 -> T_DFBlock1_K/1, T_DFBlock3_K/1, T_DFBlock2_K/1
  PHI_DFBlock2_W/1 -> Add/2
  PHI_DFBlock3_W/1 -> Add/3
  Constant1/1 -> degC->K/1(degC)
  degC->K/1(K) -> Add1/1

== system METI_TRAMI_Thermal_ver01_Jmaab_2018b_Intg/Vehicle/PTTH/DTTH_PNT/DTTH_PNT/DTTH_PNT/DFTH_PNT/DFOil2DFBlock_Heat_Resistance ==
  T_DFOil_Resi2_K : Inport
  T_DFBlock_Resi_K : Inport  Port=2
  Add : Sum  Inputs=+-
  Constant : Constant  Value=DF_PNT_DFOil2DFBlock_Heat_Resi_KpW
  Divide : Product  Inputs=*/
  Gain : Gain  Gain=-1
  Gain1 : Gain
  PHI_DFOil_Resi2_W : Outport
  PHI_DFBlock_Resi_W : Outport  Port=2
  wires:
  Constant/1 -> Divide/2
  Add/1 -> Divide/1
  Divide/1 -> Gain/1, Gain1/1
  Gain/1 -> PHI_DFOil_Resi2_W/1
  T_DFOil_Resi2_K/1 -> Add/1
  T_DFBlock_Resi_K/1 -> Add/2
  Gain1/1 -> PHI_DFBlock_Resi_W/1

== system METI_TRAMI_Thermal_ver01_Jmaab_2018b_Intg/Vehicle/PTTH/DTTH_PNT/DTTH_PNT/DTTH_PNT/DFTH_PNT/DFOil_Heat_Capacity ==
  PHI_DFOil2_W : Inport
  PHI_DFOil1_W : Inport  Port=2
  Add : Sum
  Add1 : Sum
  Constant : Constant  Value=DF_PNT_DFOil_Heat_Capa_JpK
  Constant1 : Constant  Value=DF_PNT_DFOil_Temp_ini_degC
  Divide : Product  Inputs=/*
  Integrator : Integrator
  degC->K : Subsystem
  T_DFOil2_K : Outport
  T_DFOil1_K : Outport  Port=2
  wires:
  PHI_DFOil2_W/1 -> Add/2
  PHI_DFOil1_W/1 -> Add/1
  Constant/1 -> Divide/1
  Add/1 -> Divide/2
  Divide/1 -> Integrator/1
  Integrator/1 -> Add1/2
  Add1/1 -> T_DFOil1_K/1, T_DFOil2_K/1
  Constant1/1 -> degC->K/1(degC)
  degC->K/1(K) -> Add1/1

== system METI_TRAMI_Thermal_ver01_Jmaab_2018b_Intg/Vehicle/PTTH/DTTH_PNT/DTTH_PNT/DTTH_PNT/DFTH_PNT/ENGBlock2Air_Heat_Resistance ==
  T_DFBlock_Resi_K : Inport
  T_DF_Air_Resi_K : Inport  Port=2
  Add : Sum  Inputs=+-
  Constant : Constant  Value=DF_PNT_DFBlock2DFAir_Heat_Resi_KpW
  Divide : Product  Inputs=*/
  Gain : Gain  Gain=-1
  Gain1 : Gain
  PHI_DFBlock_Resi_W : Outport
  PHI_DF_Air_Resi_W : Outport  Port=2
  wires:
  Constant/1 -> Divide/2
  Add/1 -> Divide/1
  Divide/1 -> Gain/1, Gain1/1
  Gain/1 -> PHI_DFBlock_Resi_W/1
  T_DFBlock_Resi_K/1 -> Add/1
  T_DF_Air_Resi_K/1 -> Add/2
  Gain1/1 -> PHI_DF_Air_Resi_W/1

== system METI_TRAMI_Thermal_ver01_Jmaab_2018b_Intg/Vehicle/PTTH/DTTH_PNT/DTTH_PNT/DTTH_PNT/DFTH_PNT/TMBlock2DFBlock_Heat_Resistance ==
  T_DFBlock_Resi_K : Inport
  T_TMBlock_Resi_K : Inport  Port=2
  Add : Sum  Inputs=+-
  Constant : Constant  Value=DF_PNT_TMBlock2DFBlock_Heat_Resi_KpW
  Divide : Product  Inputs=*/
  Gain : Gain  Gain=-1
  Gain1 : Gain
  PHI_DFBlock_Resi_W : Outport
  PHI_TMBlock_Resi_W : Outport  Port=2
  wires:
  Constant/1 -> Divide/2
  Add/1 -> Divide/1
  Divide/1 -> Gain/1, Gain1/1
  Gain/1 -> PHI_TMBlock_Resi_W/1
  T_TMBlock_Resi_K/1 -> Add/1
  T_DFBlock_Resi_K/1 -> Add/2
  Gain1/1 -> PHI_DFBlock_Resi_W/1

== system METI_TRAMI_Thermal_ver01_Jmaab_2018b_Intg/Vehicle/PTTH/DTTH_PNT/DTTH_PNT/DTTH_PNT/TMTH_PNT/CVTF2Coolant_Heat_Resistance ==
  note: エネルギーの
      | 向きの定義（仮）
      | ← ←←
  T_CVTF_Resi2_K : Inport
  R_CVTF_warmer_tgt_KpW : Inport  Port=2
  T_Coolant_Resi2_K : Inport  Port=3
  Add : Sum  Inputs=+-
  Divide : Product  Inputs=*/
  Gain : Gain  Gain=-1
  Gain1 : Gain  Gain=-1
  IC : InitialCondition  Value=0.1
  PHI_Coolant_Resi2_W : Outport
  PHI_CVTF_Resi2_W : Outport  Port=2
  wires:
  Add/1 -> Divide/1
  Divide/1 -> Gain/1, Gain1/1
  T_Coolant_Resi2_K/1 -> Add/2
  T_CVTF_Resi2_K/1 -> Add/1
  Gain/1 -> PHI_CVTF_Resi2_W/1
  Gain1/1 -> PHI_Coolant_Resi2_W/1
  IC/1 -> Divide/2
  R_CVTF_warmer_tgt_KpW/1 -> IC/1

== system METI_TRAMI_Thermal_ver01_Jmaab_2018b_Intg/Vehicle/PTTH/DTTH_PNT/DTTH_PNT/DTTH_PNT/TMTH_PNT/CVTF2TMBlock_Heat_Resistance ==
  T_CVTF_Resi4_K : Inport
  T_TMBlock_Resi1_K : Inport  Port=2
  Add : Sum  Inputs=+-
  Constant : Constant  Value=TM_PNT_CVTF2TMBlock_Heat_Resi_KpW
  Divide : Product  Inputs=*/
  Gain : Gain  Gain=-1
  Gain1 : Gain
  PHI_CVTF_Resi4_W : Outport
  PHI_TMBlock_Resi1_W : Outport  Port=2
  wires:
  Constant/1 -> Divide/2
  Add/1 -> Divide/1
  Divide/1 -> Gain/1, Gain1/1
  Gain/1 -> PHI_CVTF_Resi4_W/1
  T_CVTF_Resi4_K/1 -> Add/1
  T_TMBlock_Resi1_K/1 -> Add/2
  Gain1/1 -> PHI_TMBlock_Resi1_W/1

== system METI_TRAMI_Thermal_ver01_Jmaab_2018b_Intg/Vehicle/PTTH/DTTH_PNT/DTTH_PNT/DTTH_PNT/TMTH_PNT/CVTF_Heat_Capacity ==
  PHI_CVTF4_W : Inport
  PHI_CVTF1_W : Inport  Port=2
  PHI_CVT2_W : Inport  Port=3
  Add : Sum  Inputs=+++
  Add1 : Sum
  Constant : Constant  Value=TM_PNT_CVTF_Heat_Capa_JpK
  Constant1 : Constant  Value=TM_PNT_CVTF_Temp_ini_degC
  Divide : Product  Inputs=/*
  Integrator : Integrator
  degC->K : Subsystem
  T_CVTF4_K : Outport
  T_CVTF2_K : Outport  Port=2
  T_CVTF1_K : Outport  Port=3
  wires:
  PHI_CVT2_W/1 -> Add/3
  PHI_CVTF1_W/1 -> Add/1
  Constant/1 -> Divide/1
  Add/1 -> Divide/2
  Divide/1 -> Integrator/1
  Integrator/1 -> Add1/2
  Add1/1 -> T_CVTF1_K/1, T_CVTF2_K/1, T_CVTF4_K/1
  PHI_CVTF4_W/1 -> Add/2
  Constant1/1 -> degC->K/1(degC)
  degC->K/1(K) -> Add1/1

== system METI_TRAMI_Thermal_ver01_Jmaab_2018b_Intg/Vehicle/PTTH/DTTH_PNT/DTTH_PNT/DTTH_PNT/TMTH_PNT/ENGBlock2TMBlock_Heat_Resistance ==
  T_TMBlock_Resi2_K : Inport
  T_ENGBlock_Resi2_K : Inport  Port=2
  Add : Sum  Inputs=+-
  Constant : Constant  Value=TM_PNT_ENGBlock2TMBlock_Heat_Resi_KpW
  Divide : Product  Inputs=*/
  Gain : Gain  Gain=-1
  Gain1 : Gain
  PHI_TMBlock_Resi2_W : Outport
  PHI_ENGBlock_Resi2_W : Outport  Port=2
  wires:
  Constant/1 -> Divide/2
  Add/1 -> Divide/1
  Divide/1 -> Gain1/1, Gain/1
  Gain/1 -> PHI_ENGBlock_Resi2_W/1
  T_ENGBlock_Resi2_K/1 -> Add/1
  T_TMBlock_Resi2_K/1 -> Add/2
  Gain1/1 -> PHI_TMBlock_Resi2_W/1

== system METI_TRAMI_Thermal_ver01_Jmaab_2018b_Intg/Vehicle/PTTH/DTTH_PNT/DTTH_PNT/DTTH_PNT/TMTH_PNT/TMBlock2Air_Heat_Resistance ==
  T_TMBlock_Resi3_K : Inport
  T_TM_Air_Resi1_K : Inport  Port=2
  Add : Sum  Inputs=+-
  Constant : Constant  Value=TM_PNT_TMBlock2TMAir_Heat_Resi_KpW
  Divide : Product  Inputs=*/
  Gain : Gain  Gain=-1
  Gain1 : Gain
  PHI_TMBlock_Resi3_W : Outport
  PHI_TM_Air_Resi1_W : Outport  Port=2
  wires:
  Constant/1 -> Divide/2
  Add/1 -> Divide/1
  Divide/1 -> Gain/1, Gain1/1
  Gain/1 -> PHI_TMBlock_Resi3_W/1
  T_TMBlock_Resi3_K/1 -> Add/1
  T_TM_Air_Resi1_K/1 -> Add/2
  Gain1/1 -> PHI_TM_Air_Resi1_W/1

== system METI_TRAMI_Thermal_ver01_Jmaab_2018b_Intg/Vehicle/PTTH/DTTH_PNT/DTTH_PNT/DTTH_PNT/TMTH_PNT/TMBlock_Heat_Capacity ==
  PHI_TMBlock3_W : Inport
  PHI_TMBlock2_W : Inport  Port=2
  PHI_TMBlock1_W : Inport  Port=3
  PHI_TMBlock4_W : Inport  Port=4
  Add : Sum  Inputs=++++
  Add1 : Sum
  Constant : Constant  Value=TM_PNT_TMBlock_Heat_Capa_JpK
  Constant1 : Constant  Value=TM_PNT_TMBlock_Temp_ini_degC
  Divide : Product  Inputs=/*
  Integrator : Integrator
  degC->K : Subsystem
  T_TMBlock2_K : Outport
  T_TMBlock3_K : Outport  Port=2
  T_TMBlock4_K : Outport  Port=3
  T_TMBlock1_K : Outport  Port=4
  wires:
  PHI_TMBlock2_W/1 -> Add/4
  PHI_TMBlock1_W/1 -> Add/1
  Constant/1 -> Divide/1
  Add/1 -> Divide/2
  Divide/1 -> Integrator/1
  Integrator/1 -> Add1/2
  PHI_TMBlock3_W/1 -> Add/3
  PHI_TMBlock4_W/1 -> Add/2
  Add1/1 -> T_TMBlock1_K/1, T_TMBlock4_K/1, T_TMBlock3_K/1, T_TMBlock2_K/1
  Constant1/1 -> degC->K/1(degC)
  degC->K/1(K) -> Add1/1

== system METI_TRAMI_Thermal_ver01_Jmaab_2018b_Intg/Vehicle/TM_PNT/TM_PNT/TM_PNT/TM_PNT/TC_PNT/LU_Clutch ==
  note: クラッチモデル
      | LockUp ON時は硬いバネダンパー、OFF時はトルク0 Nm
  LockUP_Signal : Inport
  w_TM_PNT_in_radps1 : Inport  Port=2
  w_TM_PNT_in_radps2 : Inport  Port=3
  Gain1 : Gain  Gain=TM_PNT_Gain_LU_spring_Nmprad
  Gain2 : Gain  Gain=TM_PNT_Gain_LU_damper_Nmsprad
  Integrator : Integrator  ExternalReset=level  LimitOutput=on  UpperSaturationLimit=1  LowerSaturationLimit=-1
  Logical Operator : Logic  Operator=NOT  AllPortsSameDT=off  OutDataTypeStr=boolean
  Product : Product  RndMeth=Zero
  Product2 : Product  RndMeth=Zero
  Sum1 : Sum  Inputs=|+-
  Sum2 : Sum  Inputs=++|
  Transfer Fcn : TransferFcn  Denominator=[TM_PNT_tau_LU_Clutch_s 1]
  trq_LUC_Nm1 : Outport
  trq_LUC_Nm2 : Outport  Port=2
  wires:
  w_TM_PNT_in_radps1/1 -> Product/2
  LockUP_Signal/1 -> Logical Operator/1, Transfer Fcn/1
  Sum2/1 -> trq_LUC_Nm2/1, trq_LUC_Nm1/1
  Product2/1 -> Sum1/2
  Product/1 -> Sum1/1
  Integrator/1 -> Gain1/1
  Sum1/1 -> Integrator/1, Gain2/1
  Transfer Fcn/1 -> Product2/1, Product/1
  w_TM_PNT_in_radps2/1 -> Product2/2
  Logical Operator/1 -> Integrator/2
  Gain1/1 -> Sum2/2
  Gain2/1 -> Sum2/1

== system METI_TRAMI_Thermal_ver01_Jmaab_2018b_Intg/Vehicle/TM_PNT/TM_PNT/TM_PNT/TM_PNT/TC_PNT/T_C ==
  w_TM_PNT_in_radps1 : Inport
  w_TM_PNT_in_radps2 : Inport  Port=2
  Cal_C_Capacity : Subsystem
  Cal_Ratio_n : Subsystem
  Cal_trq_TC_eng : Subsystem
  Gain : Gain  Gain=radpsec2rpm
  Gain1 : Gain  Gain=radpsec2rpm
  Product1 : Product  RndMeth=Zero
  トルク比 Lookup Table2 : Lookup_n-D  NumberOfTableDimensions=1  BreakpointsForDimension1=TM_PNT_torque_ratio_table_x_speed_ratio  Table=TM_PNT_torque_ratio_table  ExtrapMethod=Clip  RndMeth=Simplest  InputSameDT=on
  trq_TC_Nm1 : Outport
  trq_TC_Nm2 : Outport  Port=2
  wires:
  Gain/1 -> Cal_Ratio_n/2(n_GR_rpm)  "n_GR_rpm"
  Gain1/1 -> Cal_Ratio_n/1(n_TM_PNT_rpm), Cal_trq_TC_eng/1("n_TM_PNT_rpm ")  "n_TM_PNT_rpm"
  w_TM_PNT_in_radps2/1 -> Gain/1
  Product1/1 -> trq_TC_Nm1/1
  トルク比 Lookup Table2/1 -> Product1/2
  w_TM_PNT_in_radps1/1 -> Gain1/1
  Cal_Ratio_n/1(ratio_n) -> トルク比 Lookup Table2/1, Cal_C_Capacity/1(ratio_n)
  Cal_trq_TC_eng/1(trq_TC_Nm) -> trq_TC_Nm2/1, Product1/1  "trq_TC_Nm"
  Cal_C_Capacity/1(c_capacity) -> Cal_trq_TC_eng/2(c_capacity)
  Cal_Ratio_n/2(flag_acc_del) -> Cal_C_Capacity/2(flag_acc_del)

== system METI_TRAMI_Thermal_ver01_Jmaab_2018b_Intg/Vehicle/PTTH/DTTH_PNT/DTTH_PNT/DTTH_PNT/DFTH_PNT/DFBlock_Heat_Capacity/degC->K ==
  degC : Inport
  Constant2 : Constant  Value=degC2K
  Sum : Sum  Inputs=++|
  K : Outport
  wires:
  degC/1 -> Sum/2
  Constant2/1 -> Sum/1
  Sum/1 -> K/1

== system METI_TRAMI_Thermal_ver01_Jmaab_2018b_Intg/Vehicle/PTTH/DTTH_PNT/DTTH_PNT/DTTH_PNT/DFTH_PNT/DFOil_Heat_Capacity/degC->K ==
  degC : Inport
  Constant2 : Constant  Value=degC2K
  Sum : Sum  Inputs=++|
  K : Outport
  wires:
  degC/1 -> Sum/2
  Constant2/1 -> Sum/1
  Sum/1 -> K/1

== system METI_TRAMI_Thermal_ver01_Jmaab_2018b_Intg/Vehicle/PTTH/DTTH_PNT/DTTH_PNT/DTTH_PNT/TMTH_PNT/CVTF_Heat_Capacity/degC->K ==
  degC : Inport
  Constant2 : Constant  Value=degC2K
  Sum : Sum  Inputs=++|
  K : Outport
  wires:
  degC/1 -> Sum/2
  Constant2/1 -> Sum/1
  Sum/1 -> K/1

== system METI_TRAMI_Thermal_ver01_Jmaab_2018b_Intg/Vehicle/PTTH/DTTH_PNT/DTTH_PNT/DTTH_PNT/TMTH_PNT/TMBlock_Heat_Capacity/degC->K ==
  degC : Inport
  Constant2 : Constant  Value=degC2K
  Sum : Sum  Inputs=++|
  K : Outport
  wires:
  degC/1 -> Sum/2
  Constant2/1 -> Sum/1
  Sum/1 -> K/1

== system METI_TRAMI_Thermal_ver01_Jmaab_2018b_Intg/Vehicle/TM_PNT/TM_PNT/TM_PNT/TM_PNT/TC_PNT/T_C/Cal_C_Capacity ==
  note: 容量係数
      | 加速中は＋
      | 減速中は－
  note: capacity coefficient
  note: N・m/rpm2
  ratio_n : Inport
  flag_acc_del : Inport  Port=2
  Product2 : Product  RndMeth=Zero
  ×10＾-6 : Gain  Gain=TM_PNT_ConvUnit
  容量係数 Lookup Table1 : Lookup_n-D  NumberOfTableDimensions=1  BreakpointsForDimension1=TM_PNT_torque_capacity_Nmprpm2_table_x_speed_ratio  Table=TM_PNT_torque_capacity_Nmprpm2_table  RndMeth=Simplest  InputSameDT=on
  c_capacity : Outport
  wires:
  容量係数 Lookup Table1/1 -> ×10＾-6/1
  ×10＾-6/1 -> Product2/1
  ratio_n/1 -> 容量係数 Lookup Table1/1
  Product2/1 -> c_capacity/1
  flag_acc_del/1 -> Product2/2

== system METI_TRAMI_Thermal_ver01_Jmaab_2018b_Intg/Vehicle/TM_PNT/TM_PNT/TM_PNT/TM_PNT/TC_PNT/T_C/Cal_Ratio_n ==
  n_TM_PNT_rpm : Inport
  n_GR_rpm : Inport  Port=2
  Compare To Constant1 : simulink/Logic and Bit Operations/Compare To Constant  relop=<=  const=TM_PNT_n_TC_min_rpm  OutDataTypeStr=boolean
  Compare To Constant2 : simulink/Logic and Bit Operations/Compare To Constant  relop=<=  const=TM_PNT_n_TC_min_rpm  OutDataTypeStr=boolean
  Constant : Constant  Value=0
  Logical Operator1 : Logic  Operator=OR  AllPortsSameDT=off  OutDataTypeStr=boolean
  MinMax : MinMax  Inputs=2
  Saturation1 : Saturate  UpperLimit=TM_PNT_w_ROT_T_C_UL  LowerLimit=TM_PNT_w_ROT_T_C_LL
  Saturation2 : Saturate  UpperLimit=TM_PNT_w_ROT_T_C_UL  LowerLimit=TM_PNT_w_ROT_T_C_LL
  Saturation5 : Saturate  UpperLimit=TM_PNT_ratio_w_ROT_T_C_UL  LowerLimit=TM_PNT_ratio_w_ROT_T_C_LL
  Subsystem : Subsystem
  Switch : Switch  Threshold=0.5
  加速時速度比 : Product  Inputs=*/
  減速時速度比 : Product  Inputs=*/
  ratio_n : Outport
  flag_acc_del : Outport  Port=2
  wires:
  Saturation2/1 -> 減速時速度比/1, 加速時速度比/2
  Saturation1/1 -> 減速時速度比/2, 加速時速度比/1
  加速時速度比/1 -> MinMax/1
  減速時速度比/1 -> MinMax/2
  MinMax/1 -> Saturation5/1
  Saturation5/1 -> Switch/3
  Constant/1 -> Switch/1
  Compare To Constant2/1 -> Logical Operator1/1
  Compare To Constant1/1 -> Logical Operator1/2
  Logical Operator1/1 -> Switch/2
  Switch/1 -> ratio_n/1
  n_GR_rpm/1 -> Subsystem/2(omg_tm), Saturation1/1, Compare To Constant1/1  "omg_tm"
  n_TM_PNT_rpm/1 -> Compare To Constant2/1, Subsystem/1(omg_engine), Saturation2/1  "omg_engine"
  Subsystem/1(flag_acc_del) -> flag_acc_del/1

== system METI_TRAMI_Thermal_ver01_Jmaab_2018b_Intg/Vehicle/TM_PNT/TM_PNT/TM_PNT/TM_PNT/TC_PNT/T_C/Cal_trq_TC_eng ==
  "n_TM_PNT_rpm " : Inport
  c_capacity : Inport  Port=2
  Math Function : Math  Operator=magnitude^2  SaturateOnIntegerOverflow=on
  Product : Product  RndMeth=Zero
  trq_TC_Nm : Outport
  wires:
  Product/1 -> trq_TC_Nm/1
  Math Function/1 -> Product/1
  c_capacity/1 -> Product/2
  "n_TM_PNT_rpm "/1 -> Math Function/1

== system METI_TRAMI_Thermal_ver01_Jmaab_2018b_Intg/Vehicle/TM_PNT/TM_PNT/TM_PNT/TM_PNT/TC_PNT/T_C/Cal_Ratio_n/Subsystem ==
  note: エンジン加速中は1、減速中は-1
  omg_engine : Inport
  omg_tm : Inport  Port=2
  Saturation : Saturate  UpperLimit=1  LowerLimit=-1
  Subtract : Sum  Inputs=-+|
  flag_acc_del : Outport
  wires:
  Subtract/1 -> Saturation/1
  Saturation/1 -> flag_acc_del/1
  omg_tm/1 -> Subtract/1
  omg_engine/1 -> Subtract/2
